simulink subsystem "contact_canalisation"  (R2024a)
settings: Solver=VariableStepAuto  StartTime=0.0  StopTime=10.0  RelTol=1e-3
libraries: nesl_utility x24, sm_lib x12
settings Model: Creator=Acwa-Remote  LastModifiedBy=VincentPERRET

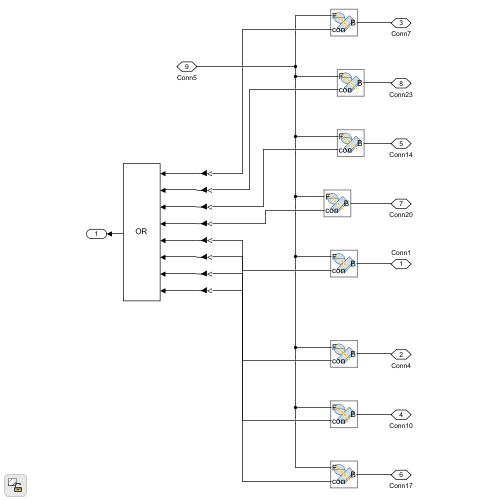
[thumbnail: Simulink's stored preview of the top-level diagram]
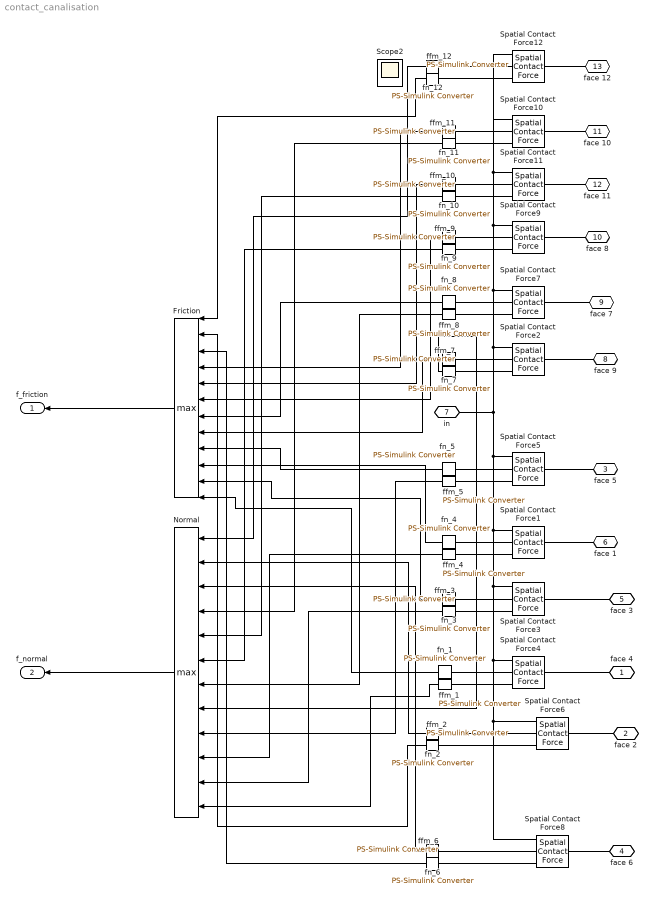
== system contact_canalisation ==
  Friction : MinMax  Function=max  Inputs=12
  Normal : MinMax  Function=max  Inputs=12
  Scope2 : Scope  NumInputPorts=2
  Spatial Contact Force{1..7,9..12} (11 alike) : sm_lib/Forces and Torques/Spatial Contact Force  NormalForceType=SmoothSpringDamper  NormalStiffness=stiff  NormalStiffnessUnits=N/m  NormalDamping=damp  NormalDampingUnits=N/(m/s)  NormalTransitionRegionWidth=trw  NormalTransitionRegionWidthUnits=mm  FrictionType=SmoothStickSlip  CoefficientOfStaticFriction=cana_fs  CoefficientOfDynamicFriction=cana_fd  FrictionalCriticalVelocity=1e-3  FrictionalCriticalVelocityUnits=m/s  SenseContactSignal=off  SensePenetrationDepth=off  SenseSeparationDistance=off  SenseNormalForceMagnitude=on  SenseFrictionalForceMagnitude=on  SenseNormalVelocity=off  SenseTangentialVelocity=off  SenseContactBaseRotation=off  SenseContactBaseTranslation=off  SenseContactFollowerRotation=off  SenseContactFollowerTranslation=off  ZeroCrossDetectContactStartAndEnd=off
  Spatial Contact Force8 : sm_lib/Forces and Torques/Spatial Contact Force  NormalForceType=SmoothSpringDamper  NormalStiffness=stiff  NormalStiffnessUnits=N/m  NormalDamping=damp  NormalDampingUnits=N/(m/s)  NormalTransitionRegionWidth=trw  NormalTransitionRegionWidthUnits=mm  FrictionType=SmoothStickSlip  CoefficientOfStaticFriction=0.3  CoefficientOfDynamicFriction=0.3  FrictionalCriticalVelocity=1e-3  FrictionalCriticalVelocityUnits=m/s  SenseContactSignal=off  SensePenetrationDepth=off  SenseSeparationDistance=off  SenseNormalForceMagnitude=on  SenseFrictionalForceMagnitude=on  SenseNormalVelocity=off  SenseTangentialVelocity=off  SenseContactBaseRotation=off  SenseContactBaseTranslation=off  SenseContactFollowerRotation=off  SenseContactFollowerTranslation=off  ZeroCrossDetectContactStartAndEnd=off
  ffm_{1..12} (12 alike) : nesl_utility/PS-Simulink Converter  PhysicalDomain=network_engine_domain  SubClassName=ps_output  LeftPortType=input  RightPortType=output  PseudoPeriodic=off  Frequencies=[]  VectorFormat=inherit  Unit=inherit  AffineConversion=off
  fn_{1..12} (12 alike) : nesl_utility/PS-Simulink Converter  PhysicalDomain=network_engine_domain  SubClassName=ps_output  LeftPortType=input  RightPortType=output  PseudoPeriodic=off  Frequencies=[]  VectorFormat=inherit  Unit=inherit  AffineConversion=off
  face 4 : PMIOPort  Side=Left
  face 2 : PMIOPort  Port=2  Side=Left
  face 5 : PMIOPort  Port=3  Side=Left
  face 6 : PMIOPort  Port=4  Side=Left
  face 3 : PMIOPort  Port=5  Side=Left
  face 1 : PMIOPort  Port=6  Side=Left
  in : PMIOPort  Port=7  Side=Right
  face 9 : PMIOPort  Port=8  Side=Left
  face 7 : PMIOPort  Port=9  Side=Left
  face 8 : PMIOPort  Port=10  Side=Left
  face 10 : PMIOPort  Port=11  Side=Left
  face 11 : PMIOPort  Port=12  Side=Left
  face 12 : PMIOPort  Port=13  Side=Left
  f_friction : Outport
  f_normal : Outport  Port=2
  wires:
  fn_2/1 -> Normal/2
  ffm_2/1 -> Friction/2
  ffm_6/1 -> Friction/3
  fn_6/1 -> Normal/3
  ffm_12/1 -> Friction/1
  fn_12/1 -> Normal/1
  Friction/1 -> f_friction/1
  Normal/1 -> f_normal/1
  fn_11/1 -> Friction/4
  fn_10/1 -> Friction/5
  fn_9/1 -> Friction/6
  fn_8/1 -> Friction/7
  fn_7/1 -> Friction/8
  fn_5/1 -> Friction/9
  fn_4/1 -> Friction/10
  fn_3/1 -> Friction/11
  fn_1/1 -> Friction/12
  ffm_11/1 -> Normal/4
  ffm_10/1 -> Normal/5
  ffm_9/1 -> Normal/6
  ffm_8/1 -> Normal/7
  ffm_7/1 -> Normal/8
  ffm_5/1 -> Normal/9
  ffm_4/1 -> Normal/10
  ffm_3/1 -> Normal/11
  ffm_1/1 -> Normal/12
  connections:
  Spatial Contact Force8/RConn1 -- Spatial Contact Force5/RConn1 -- in/RConn1 -- Spatial Contact Force2/RConn1 -- Spatial Contact Force7/RConn1 -- Spatial Contact Force9/RConn1 -- Spatial Contact Force11/RConn1 -- Spatial Contact Force10/RConn1 -- Spatial Contact Force12/RConn1 -- Spatial Contact Force1/RConn1 -- Spatial Contact Force3/RConn1 -- Spatial Contact Force4/RConn1 -- Spatial Contact Force6/RConn1
  face 1/RConn1 -- Spatial Contact Force1/LConn1
  Spatial Contact Force6/RConn2 -- fn_2/LConn1
  ffm_6/LConn1 -- Spatial Contact Force8/RConn3
  Spatial Contact Force5/LConn1 -- face 5/RConn1
  Spatial Contact Force3/LConn1 -- face 3/RConn1
  Spatial Contact Force4/LConn1 -- face 4/RConn1
  Spatial Contact Force6/LConn1 -- face 2/RConn1
  Spatial Contact Force8/LConn1 -- face 6/RConn1
  Spatial Contact Force2/LConn1 -- face 9/RConn1
  Spatial Contact Force7/LConn1 -- face 7/RConn1
  Spatial Contact Force9/LConn1 -- face 8/RConn1
  Spatial Contact Force10/LConn1 -- face 10/RConn1
  Spatial Contact Force12/RConn3 -- ffm_12/LConn1
  Spatial Contact Force11/LConn1 -- face 11/RConn1
  Spatial Contact Force12/LConn1 -- face 12/RConn1
  fn_12/LConn1 -- Spatial Contact Force12/RConn2
  ffm_2/LConn1 -- Spatial Contact Force6/RConn3
  fn_6/LConn1 -- Spatial Contact Force8/RConn2
  fn_1/LConn1 -- Spatial Contact Force4/RConn2
  ffm_1/LConn1 -- Spatial Contact Force4/RConn3
  fn_3/LConn1 -- Spatial Contact Force3/RConn2
  ffm_3/LConn1 -- Spatial Contact Force3/RConn3
  ffm_4/LConn1 -- Spatial Contact Force1/RConn3
  fn_4/LConn1 -- Spatial Contact Force1/RConn2
  fn_5/LConn1 -- Spatial Contact Force5/RConn2
  ffm_5/LConn1 -- Spatial Contact Force5/RConn3
  fn_7/LConn1 -- Spatial Contact Force2/RConn2
  ffm_7/LConn1 -- Spatial Contact Force2/RConn3
  fn_8/LConn1 -- Spatial Contact Force7/RConn2
  ffm_8/LConn1 -- Spatial Contact Force7/RConn3
  fn_9/LConn1 -- Spatial Contact Force9/RConn2
  ffm_9/LConn1 -- Spatial Contact Force9/RConn3
  fn_10/LConn1 -- Spatial Contact Force11/RConn2
  ffm_10/LConn1 -- Spatial Contact Force11/RConn3
  fn_11/LConn1 -- Spatial Contact Force10/RConn2
  ffm_11/LConn1 -- Spatial Contact Force10/RConn3
